simulink model "ftc_ut"  (Simulink 8.1)
settings: Solver=FixedStepDiscrete  StartTime=0.0  StopTime=Inf  FixedStep=0.005  RelTol=1e-3
undefined symbols (not defined in the file or in its folder): Calculation_of_FCW_Last_Point_to_Brake, ftc, KJUD_DecelThreshBraking_mps2, KJUD_FCWConsideredDecel_mps2
libraries: fhfr x1, pbnbs x1, pbbs_new x1
settings Model: Creator=xsellart  LastModifiedBy=AT015555
settings DataIOCC: SignalLoggingSaveFormat=Dataset
settings OptimizationCC: ExpressionDepthLimit=128
settings DebuggingCC: FcnCallInpInsideContextMsg=EnableAllAsError
settings GRTTargetCC: CombineOutputUpdateFcns=on  GRTInterface=off

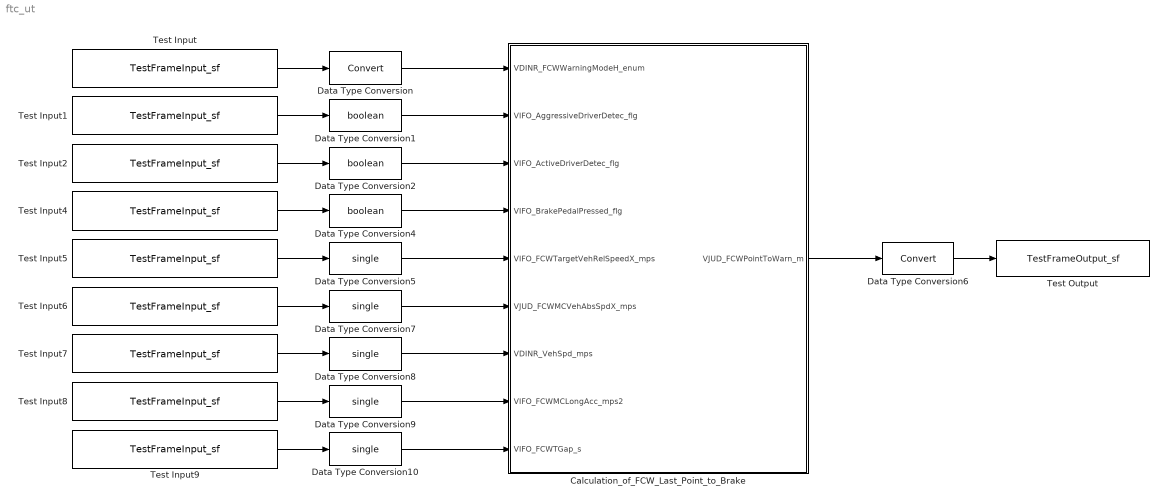
== system ftc_ut ==
  Calculation_of_FCW_Last_Point_to_Brake : Subsystem  AncestorBlock=ftc/Calculation_of_FCW_Last_Point_to_Brake
  Data Type Conversion : DataTypeConversion
  Data Type Conversion1 : DataTypeConversion  OutDataTypeStr=boolean
  Data Type Conversion{5,7..10} (5 alike) : DataTypeConversion  OutDataTypeStr=single
  Data Type Conversion2 : DataTypeConversion  OutDataTypeStr=boolean
  Data Type Conversion4 : DataTypeConversion  OutDataTypeStr=boolean
  Data Type Conversion6 : DataTypeConversion
  Test Input : S-Function  FunctionName=TestFrameInput_sf  Parameters=varname,sampletime  EnableBusSupport=off  mask(Test Input){varname=VDINR_FCWWarningModeH_enum, sampletime=0.005}
      mask prompts: varname "Name:"; sampletime "Sample Time:"
      mask help: Outputs the value of a Test Input variable from an Excel spreadsheet when used with the runsiltest script. Otherwise outputs 0.
      mask Display: fprintf('Test Input:\n%s',varname);
  Test Input1 : S-Function  FunctionName=TestFrameInput_sf  Parameters=varname,sampletime  EnableBusSupport=off  mask(Test Input){varname=VIFO_AggressiveDriverDetec_flg, sampletime=0.005}
      mask prompts: varname "Name:"; sampletime "Sample Time:"
      mask help: Outputs the value of a Test Input variable from an Excel spreadsheet when used with the runsiltest script. Otherwise outputs 0.
      mask Display: fprintf('Test Input:\n%s',varname);
  Test Input2 : S-Function  FunctionName=TestFrameInput_sf  Parameters=varname,sampletime  EnableBusSupport=off  mask(Test Input){varname=VIFO_ActiveDriverDetec_flg, sampletime=0.005}
      mask prompts: varname "Name:"; sampletime "Sample Time:"
      mask help: Outputs the value of a Test Input variable from an Excel spreadsheet when used with the runsiltest script. Otherwise outputs 0.
      mask Display: fprintf('Test Input:\n%s',varname);
  Test Input4 : S-Function  FunctionName=TestFrameInput_sf  Parameters=varname,sampletime  EnableBusSupport=off  mask(Test Input){varname=VIFO_BrakePedalPressed_flg, sampletime=0.005}
      mask prompts: varname "Name:"; sampletime "Sample Time:"
      mask help: Outputs the value of a Test Input variable from an Excel spreadsheet when used with the runsiltest script. Otherwise outputs 0.
      mask Display: fprintf('Test Input:\n%s',varname);
  Test Input5 : S-Function  FunctionName=TestFrameInput_sf  Parameters=varname,sampletime  EnableBusSupport=off  mask(Test Input){varname=VIFO_FCWTargetVehRelSpeedX_mps, sampletime=0.005}
      mask prompts: varname "Name:"; sampletime "Sample Time:"
      mask help: Outputs the value of a Test Input variable from an Excel spreadsheet when used with the runsiltest script. Otherwise outputs 0.
      mask Display: fprintf('Test Input:\n%s',varname);
  Test Input6 : S-Function  FunctionName=TestFrameInput_sf  Parameters=varname,sampletime  EnableBusSupport=off  mask(Test Input){varname=VJUD_FCWMCVehAbsSpdX_mps, sampletime=0.005}
      mask prompts: varname "Name:"; sampletime "Sample Time:"
      mask help: Outputs the value of a Test Input variable from an Excel spreadsheet when used with the runsiltest script. Otherwise outputs 0.
      mask Display: fprintf('Test Input:\n%s',varname);
  Test Input7 : S-Function  FunctionName=TestFrameInput_sf  Parameters=varname,sampletime  EnableBusSupport=off  mask(Test Input){varname=VDINR_VehSpd_mps, sampletime=0.005}
      mask prompts: varname "Name:"; sampletime "Sample Time:"
      mask help: Outputs the value of a Test Input variable from an Excel spreadsheet when used with the runsiltest script. Otherwise outputs 0.
      mask Display: fprintf('Test Input:\n%s',varname);
  Test Input8 : S-Function  FunctionName=TestFrameInput_sf  Parameters=varname,sampletime  EnableBusSupport=off  mask(Test Input){varname=VIFO_FCWMCLongAcc_mps2, sampletime=0.005}
      mask prompts: varname "Name:"; sampletime "Sample Time:"
      mask help: Outputs the value of a Test Input variable from an Excel spreadsheet when used with the runsiltest script. Otherwise outputs 0.
      mask Display: fprintf('Test Input:\n%s',varname);
  Test Input9 : S-Function  FunctionName=TestFrameInput_sf  Parameters=varname,sampletime  EnableBusSupport=off  mask(Test Input){varname=VIFO_FCWTGap_s, sampletime=0.005}
      mask prompts: varname "Name:"; sampletime "Sample Time:"
      mask help: Outputs the value of a Test Input variable from an Excel spreadsheet when used with the runsiltest script. Otherwise outputs 0.
      mask Display: fprintf('Test Input:\n%s',varname);
  Test Output : S-Function  FunctionName=TestFrameOutput_sf  Parameters=varname,sampletime  EnableBusSupport=off  mask(Test Output){varname=VJUD_FCWPointToWarn_m, sampletime=-1}
      mask prompts: varname "Name:"; sampletime "Sample Time:"
      mask help: Samples the value of a Test Output variable from an Excel spreadsheet when used with the runsiltest script. Otherwise does nothing.
      mask Display: fprintf('Test Output:\n%s',varname);
  wires:
  Test Input/1 -> Data Type Conversion/1
  Data Type Conversion/1 -> Calculation_of_FCW_Last_Point_to_Brake/1(VDINR_FCWWarningModeH_enum)
  Test Input1/1 -> Data Type Conversion1/1
  Data Type Conversion1/1 -> Calculation_of_FCW_Last_Point_to_Brake/2(VIFO_AggressiveDriverDetec_flg)
  Test Input2/1 -> Data Type Conversion2/1
  Calculation_of_FCW_Last_Point_to_Brake/1(VJUD_FCWPointToWarn_m) -> Data Type Conversion6/1
  Data Type Conversion6/1 -> Test Output/1
  Data Type Conversion2/1 -> Calculation_of_FCW_Last_Point_to_Brake/3(VIFO_ActiveDriverDetec_flg)
  Test Input4/1 -> Data Type Conversion4/1
  Data Type Conversion4/1 -> Calculation_of_FCW_Last_Point_to_Brake/4(VIFO_BrakePedalPressed_flg)
  Test Input5/1 -> Data Type Conversion5/1
  Data Type Conversion5/1 -> Calculation_of_FCW_Last_Point_to_Brake/5(VIFO_FCWTargetVehRelSpeedX_mps)
  Test Input6/1 -> Data Type Conversion7/1
  Data Type Conversion7/1 -> Calculation_of_FCW_Last_Point_to_Brake/6(VJUD_FCWMCVehAbsSpdX_mps)
  Test Input7/1 -> Data Type Conversion8/1
  Data Type Conversion8/1 -> Calculation_of_FCW_Last_Point_to_Brake/7(VDINR_VehSpd_mps)
  Test Input8/1 -> Data Type Conversion9/1
  Data Type Conversion9/1 -> Calculation_of_FCW_Last_Point_to_Brake/8(VIFO_FCWMCLongAcc_mps2)
  Test Input9/1 -> Data Type Conversion10/1
  Data Type Conversion10/1 -> Calculation_of_FCW_Last_Point_to_Brake/9(VIFO_FCWTGap_s)

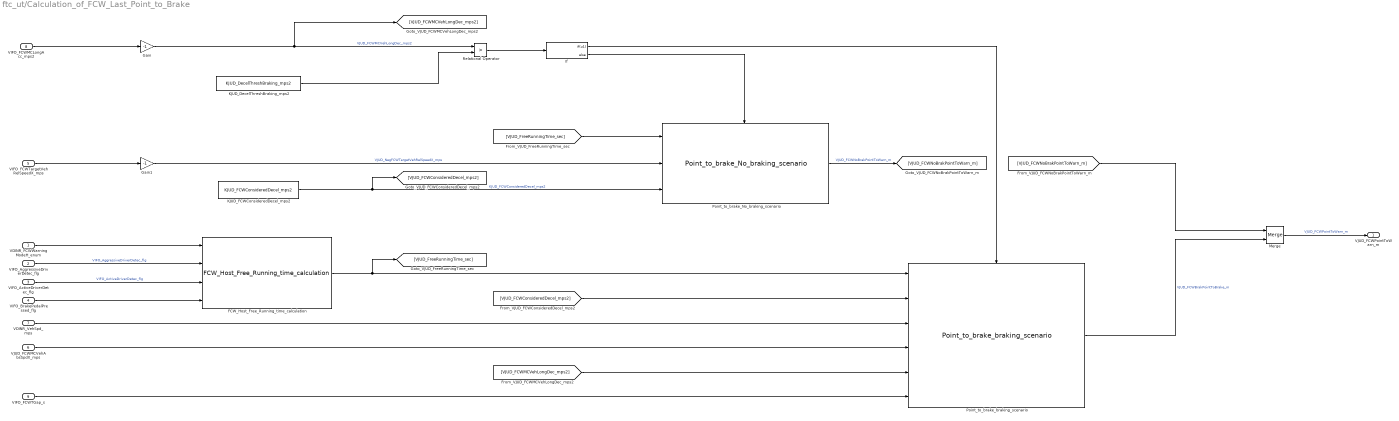
== system ftc_ut/Calculation_of_FCW_Last_Point_to_Brake ==
  VDINR_FCWWarningModeH_enum : Inport
  VIFO_AggressiveDriverDetec_flg : Inport  Port=2
  VIFO_ActiveDriverDetec_flg : Inport  Port=3
  VIFO_BrakePedalPressed_flg : Inport  Port=4
  VIFO_FCWTargetVehRelSpeedX_mps : Inport  Port=5
  VJUD_FCWMCVehAbsSpdX_mps : Inport  Port=6
  VDINR_VehSpd_mps : Inport  Port=7
  VIFO_FCWMCLongAcc_mps2 : Inport  Port=8
  VIFO_FCWTGap_s : Inport  Port=9
  FCW_Host_Free_Running_time_calculation : fhfr/FCW_Host_Free_Running_time_calculation
  Gain : Gain  Gain=-1  OutDataTypeStr=single
  Gain1 : Gain  Gain=-1  OutDataTypeStr=single
  If : If  IfExpression=u1
  KJUD_DecelThreshBraking_mps2 : Constant  Value=KJUD_DecelThreshBraking_mps2  OutDataTypeStr=single
  KJUD_FCWConsideredDecel_mps2 : Constant  Value=KJUD_FCWConsideredDecel_mps2
  Merge : Merge
  Point_to_brake_No_braking_scenario : pbnbs/Point_to_brake_No_braking_scenario
  Point_to_brake_braking_scenario : pbbs_new/Point_to_brake_braking_scenario
  Relational Operator : RelationalOperator  Operator=>  OutDataTypeStr=boolean
  VJUD_FCWPointToWarn_m : Outport
  wires:
  VIFO_FCWTGap_s/1 -> Point_to_brake_braking_scenario/6
  VDINR_FCWWarningModeH_enum/1 -> FCW_Host_Free_Running_time_calculation/1
  Merge/1 -> VJUD_FCWPointToWarn_m/1  "VJUD_FCWPointToWarn_m"
  Point_to_brake_braking_scenario/1 -> Merge/2  "VJUD_FCWBrakPointToBrake_m"
  [VJUD_FCWNoBrakPointToWarn_m] -> Merge/1
  Point_to_brake_No_braking_scenario/1 -> [VJUD_FCWNoBrakPointToWarn_m]  "VJUD_FCWNoBrakPointToWarn_m"
  If/2 -> Point_to_brake_No_braking_scenario/Action
  KJUD_FCWConsideredDecel_mps2/1 -> Point_to_brake_No_braking_scenario/3, [VJUD_FCWConsideredDecel_mps2]  "KJUD_FCWConsideredDecel_mps2"
  Gain1/1 -> Point_to_brake_No_braking_scenario/2  "VJUD_NegFCWTargetVehRelSpeedX_mps"
  [VJUD_FreeRunningTime_sec] -> Point_to_brake_No_braking_scenario/1
  [VJUD_FCWMCVehLongDec_mps2] -> Point_to_brake_braking_scenario/5
  If/1 -> Point_to_brake_braking_scenario/Action
  FCW_Host_Free_Running_time_calculation/1 -> Point_to_brake_braking_scenario/1, [VJUD_FreeRunningTime_sec]
  VJUD_FCWMCVehAbsSpdX_mps/1 -> Point_to_brake_braking_scenario/4
  [VJUD_FCWConsideredDecel_mps2] -> Point_to_brake_braking_scenario/2
  VDINR_VehSpd_mps/1 -> Point_to_brake_braking_scenario/3
  Relational Operator/1 -> If/1
  Gain/1 -> Relational Operator/1, [VJUD_FCWMCVehLongDec_mps2]  "VJUD_FCWMCVehLongDec_mps2"
  VIFO_FCWTargetVehRelSpeedX_mps/1 -> Gain1/1
  KJUD_DecelThreshBraking_mps2/1 -> Relational Operator/2
  VIFO_FCWMCLongAcc_mps2/1 -> Gain/1
  VIFO_BrakePedalPressed_flg/1 -> FCW_Host_Free_Running_time_calculation/4
  VIFO_ActiveDriverDetec_flg/1 -> FCW_Host_Free_Running_time_calculation/3  "VIFO_ActiveDriverDetec_flg"
  VIFO_AggressiveDriverDetec_flg/1 -> FCW_Host_Free_Running_time_calculation/2  "VIFO_AggressiveDriverDetec_flg"
